simulink model "vehicle_longitudinal_model"  (R2021a)
settings: Solver=VariableStepAuto  StartTime=0.0  StopTime=10.0  RelTol=1e-3
InitFcn:
  | %{
  | Adv Powertrain Modeling HW#3
  | Written By: Matt Asper
  | Date: 2023 Feb 16
  | 
  | This project is a vehicle longitudinal model
  | with electric motor for a concept vehicle.
  | %}
  | 
  | clc; clear; close all;
  | 
  | cd('/Users/asper101/Library/CloudStorage/OneDrive-Personal/Grad School/Advanced Powertrain Modeling/HWs/HW3')
  | 
  | vehicle_longitudinal_para
  | 
  | %inputs
  | T0 = 0; %starting throttle
  | Tf = 100; %ending throttle
  | B = 25; %break magnitude
  | alpha = 5; %incline angle (deg)
  | v0 = 20; %initial velocity (m/s)
  | wg0 = 0; %initial MG1 angular velocity (rad/s)
values from neighbouring files (symbols this model uses):
  A_front = 9.5    [VehicleLongtitudinalModel.m]    (also in vehicle_longitudinal_para.m)
  Cd = 0.7963    [VehicleLongtitudinalModel.m]    (also in vehicle_longitudinal_para.m)
  Cr = 0.0085    [VehicleLongtitudinalModel.m]    (also in vehicle_longitudinal_para.m)
  eng_consum_fuel = [0 0 0 0 0 0 0 0 0 0 0 0 ... (1220 elements, 61x20)]    [eng_consum_fuel.mat]    (also in vehicle_longitudinal_para.m = eng_consum_fuel * 6)
  eng_consum_spd = [52.35 55 57.6 60.2 62.85 65.45 68.05 70.7 73.3 75.9 78.55 81.15 ... (61 elements, 1x61)]    [eng_consum_fuel.mat]    (also in vehicle_longitudinal_para.m = eng_consum_spd / 2)
  eng_consum_trq = [0 137.659783677 206.489675516 275.319567355 344.149459194 412.979351032 481.809242871 550.63913471 619.469026549 688.298918387 757.128810226 825.958702065 ... (20 elements, 1x20)]    [eng_consum_fuel.mat]    (also in vehicle_longitudinal_para.m = eng_consum_trq * (1400 / 1.356 / 75))
  eng_map_fuel = [0 0.1 0.2 0.3 0.4 0.5 0.6 0.7 0.8 0.9 1]    [eng_consum_fuel.mat]    (also in vehicle_longitudinal_para.m)
  eng_map_spd = [52.35 55 57.6 60.2 62.85 65.45 68.05 70.7 73.3 75.9 78.55 81.15 ... (61 elements, 1x61)]    [eng_consum_fuel.mat]    (also in vehicle_longitudinal_para.m = eng_map_spd * (2000 / 4000))
  eng_map_trq = [0 106.452310718 212.904621436 319.356932153 425.809242871 532.261553589 638.713864307 745.166175025 851.618485742 958.07079646 1064.52310718 0 ... (671 elements, 11x61)]    [eng_consum_fuel.mat]    (also in vehicle_longitudinal_para.m = zeros(length(eng_map_fuel), length(eng_map_spd)))
  FR = 1.18    [VehicleLongtitudinalModel.m]    (also in vehicle_longitudinal_para.m)
  g = 9.81    [VehicleLongtitudinalModel.m]    (also in vehicle_longitudinal_para.m)
  Ic = 0    [VehicleLongtitudinalModel.m]    (also in vehicle_longitudinal_para.m)
  Ie = e_inertia    (= 1.8)    [vehicle_longitudinal_para.m]
  Ig = g_inertia    (= 0.0226)    [vehicle_longitudinal_para.m]
  Im = m_inertia    (= 0.226)    [vehicle_longitudinal_para.m]
  Ir = 0    [VehicleLongtitudinalModel.m]    (also in vehicle_longitudinal_para.m)
  Is = 0    [VehicleLongtitudinalModel.m]    (also in vehicle_longitudinal_para.m)
  m_eff_map = [0.85975 0.532 0.684 0.684 0.684 0.684 0.684 0.684 0.684 0.684 0.684 0.85975 ... (253 elements, 11x23)]    [m_eff_map.mat]    (also in vehicle_longitudinal_para.m = 0.95*[ .905    .905    .905    .905    .905    .905    .905 )
  m_map_spd = [0 52.3598775598 104.71975512 157.079632679 209.439510239 261.799387799 314.159265359 366.519142919 418.879020479 471.238898038 628.318530718]    [m_eff_map.mat]    (also in vehicle_longitudinal_para.m = [0 500 1000 1500 2000 2500 3000 3500 4000 4500 6000]*(2*pi)/)
  m_map_trq = [-2033.33333333 -1833.33333333 -1633.33333333 -1433.33333333 -1233.33333333 -1033.33333333 -833.333333333 -633.333333333 -433.333333333 -233.333333333 -33.3333333333 0 ... (23 elements, 1x23)]    [m_eff_map.mat]    (also in vehicle_longitudinal_para.m = m_map_trq * (200 / 30))
  N = 4    [vehicle_longitudinal_para.m]
  Nr = 78    [VehicleLongtitudinalModel.m]    (also in vehicle_longitudinal_para.m)
  Ns = 30    [VehicleLongtitudinalModel.m]    (also in vehicle_longitudinal_para.m)
  R_tire = 0.5    [VehicleLongtitudinalModel.m]    (also in vehicle_longitudinal_para.m)
  rho_air = 1.2    [VehicleLongtitudinalModel.m]    (also in vehicle_longitudinal_para.m)
  Vehicle_mass = 15076    [VehicleLongtitudinalModel.m]    (also in vehicle_longitudinal_para.m)
settings Model: Creator=asper101  LastModifiedBy=asper101

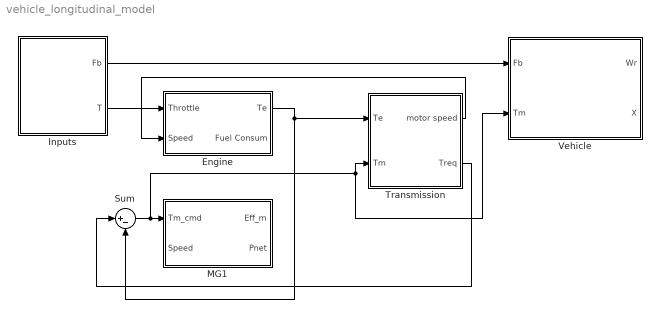
== system vehicle_longitudinal_model ==
  Engine : Subsystem
  Inputs : Subsystem
  MG1 : Subsystem
  Sum : Sum  Inputs=|+-
  Transmission : Subsystem
  Vehicle : Subsystem
  wires:
  Inputs/2(T) -> Engine/1(Throttle)
  Transmission/1(motor speed) -> Engine/2(Speed)
  Engine/1(Te) -> Transmission/1(Te), Sum/2
  Transmission/2(Treq) -> Sum/1
  Sum/1 -> Vehicle/2(Tm), Transmission/2(Tm), MG1/1(Tm_cmd)
  Inputs/1(Fb) -> Vehicle/1(Fb)

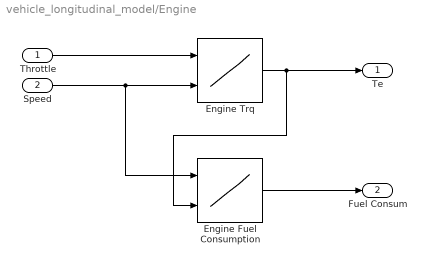
== system vehicle_longitudinal_model/Engine ==
  Throttle : Inport
  Speed : Inport  Port=2
  Engine Fuel Consumption : Lookup_n-D  BreakpointsForDimension1=eng_consum_spd  BreakpointsForDimension2=eng_consum_trq  Table=eng_consum_fuel  InternalRulePriority=Speed  RndMeth=Simplest  InputSameDT=on
      settings: InputPortMap=u0,u1
  Engine Trq : Lookup_n-D  BreakpointsForDimension1=eng_map_fuel  BreakpointsForDimension2=eng_map_spd  Table=eng_map_trq  InternalRulePriority=Speed  RndMeth=Simplest  InputSameDT=on
      settings: InputPortMap=u0,u1
  Te : Outport
  Fuel Consum : Outport  Port=2
  wires:
  Throttle/1 -> Engine Trq/1
  Speed/1 -> Engine Fuel Consumption/1, Engine Trq/2
  Engine Fuel Consumption/1 -> Fuel Consum/1
  Engine Trq/1 -> Te/1, Engine Fuel Consumption/2

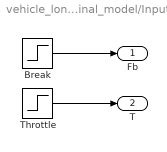
== system vehicle_longitudinal_model/Inputs ==
  Break : Step  Time=5  After=B  SampleTime=0
  Throttle : Step  Before=T0  After=Tf  SampleTime=0
  Fb : Outport
  T : Outport  Port=2
  wires:
  Throttle/1 -> T/1
  Break/1 -> Fb/1

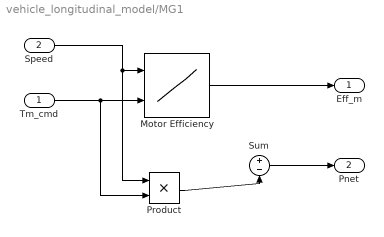
== system vehicle_longitudinal_model/MG1 ==
  Tm_cmd : Inport
  Speed : Inport  Port=2
  Motor Efficiency : Lookup_n-D  BreakpointsForDimension1=m_map_spd  BreakpointsForDimension2=m_map_trq  Table=m_eff_map  InternalRulePriority=Speed  RndMeth=Simplest  InputSameDT=on
      settings: InputPortMap=u0,u1
  Product : Product
  Sum : Sum  Inputs=+-
  Eff_m : Outport
  Pnet : Outport  Port=2
  wires:
  Motor Efficiency/1 -> Eff_m/1
  Speed/1 -> Product/1, Motor Efficiency/1
  Tm_cmd/1 -> Product/2, Motor Efficiency/2
  Product/1 -> Sum/2
  Sum/1 -> Pnet/1

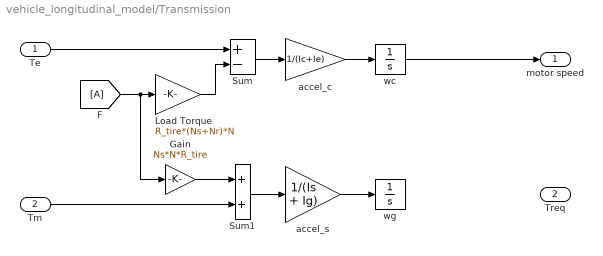
== system vehicle_longitudinal_model/Transmission ==
  Te : Inport
  Tm : Inport  Port=2
  Gain : Gain  Gain=Ns*N*R_tire
  Load Torque : Gain  Gain=R_tire*(Ns+Nr)*N
  Sum : Sum  Inputs=+-
  Sum1 : Sum
  accel_c : Gain  Gain=1/(Ic+Ie)
  accel_s : Gain  Gain=1/(Is + Ig)
  wc : Integrator  InitialCondition=(v0/R_tire*2*pi*Nr + wg0*Ns)/(Nr + Ns)
  wg : Integrator  InitialCondition=wg0
  motor speed : Outport
  Treq : Outport  Port=2
  wires:
  Te/1 -> Sum/1
  [A] -> Gain/1, Load Torque/1
  Load Torque/1 -> Sum/2
  Sum/1 -> accel_c/1
  accel_c/1 -> wc/1
  Gain/1 -> Sum1/1
  Tm/1 -> Sum1/2
  Sum1/1 -> accel_s/1
  accel_s/1 -> wg/1
  wc/1 -> motor speed/1

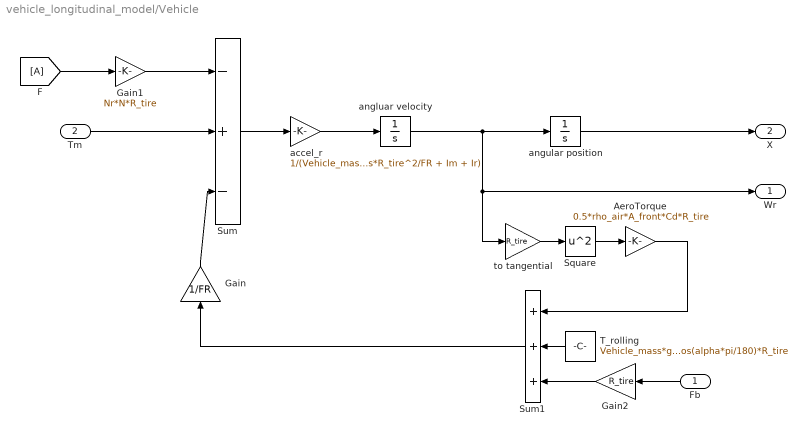
== system vehicle_longitudinal_model/Vehicle ==
  Fb : Inport
  Tm : Inport  Port=2
  AeroTorque : Gain  Gain=0.5*rho_air*A_front*Cd*R_tire
  Gain : Gain  Gain=1/FR
  Gain1 : Gain  Gain=Nr*N*R_tire
  Gain2 : Gain  Gain=R_tire
  Square : Math  Operator=square  SaturateOnIntegerOverflow=on
  Sum : Sum  Inputs=-+-
  Sum1 : Sum  Inputs=+++
  T_rolling : Constant  Value=Vehicle_mass*g*Cr*cos(alpha*pi/180)*R_tire
  accel_r : Gain  Gain=1/(Vehicle_mass*R_tire^2/FR + Im + Ir)
  angluar velocity : Integrator  InitialCondition=v0/R_tire*2*pi
  angular position : Integrator
  to tangential : Gain  Gain=R_tire
  Wr : Outport
  X : Outport  Port=2
  wires:
  angluar velocity/1 -> angular position/1, Wr/1, to tangential/1
  Square/1 -> AeroTorque/1
  to tangential/1 -> Square/1
  T_rolling/1 -> Sum1/2
  AeroTorque/1 -> Sum1/1
  Sum1/1 -> Gain/1
  Tm/1 -> Sum/2
  Sum/1 -> accel_r/1
  accel_r/1 -> angluar velocity/1
  angular position/1 -> X/1
  Gain/1 -> Sum/3
  Gain1/1 -> Sum/1
  [A] -> Gain1/1
  Fb/1 -> Gain2/1
  Gain2/1 -> Sum1/3
